simulink library "INT_CnvSet_Trq2Q"  (R2016b)
settings: Solver=VariableStepAuto  StartTime=0.0  StopTime=10.0  RelTol=1e-3
settings Model: Creator=xuxingpei  LastModifiedBy=xuxingpei

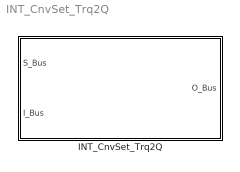
== system INT_CnvSet_Trq2Q ==
  INT_CnvSet_Trq2Q : Subsystem

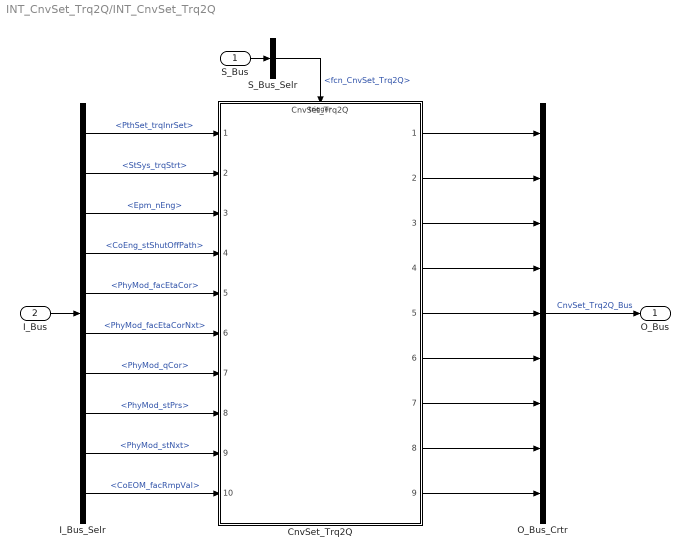
== system INT_CnvSet_Trq2Q/INT_CnvSet_Trq2Q ==
  S_Bus : Inport
  I_Bus : Inport  Port=2
  CnvSet_Trq2Q : ModelReference  ModelNameDialog=CnvSet_Trq2Q  SimulationMode=Normal  ModelReferenceVersion=1.57  TriggerPortName=function  TriggerPortTriggerType=function-call  TriggerPortStatesWhenEnabling=held
  I_Bus_Selr : BusSelector  OutputSignals=PthSet_trqInrSet,StSys_trqStrt,Epm_nEng,CoEng_stShutOffPath,PhyMod_facEtaCor,PhyMod_facEtaCorNxt,PhyMod_qCor,PhyMod_stPrs,PhyMod_stNxt,CoEOM_facRmpVal
  O_Bus_Crtr : BusCreator  Inputs=9
  S_Bus_Selr : BusSelector  OutputSignals=fcn_CnvSet_Trq2Q
  O_Bus : Outport
  wires:
  S_Bus_Selr/1 -> CnvSet_Trq2Q/Trigger  "<fcn_CnvSet_Trq2Q>"
  S_Bus/1 -> S_Bus_Selr/1
  I_Bus/1 -> I_Bus_Selr/1
  I_Bus_Selr/1 -> CnvSet_Trq2Q/1  "<PthSet_trqInrSet>"
  I_Bus_Selr/2 -> CnvSet_Trq2Q/2  "<StSys_trqStrt>"
  I_Bus_Selr/3 -> CnvSet_Trq2Q/3  "<Epm_nEng>"
  I_Bus_Selr/4 -> CnvSet_Trq2Q/4  "<CoEng_stShutOffPath>"
  I_Bus_Selr/5 -> CnvSet_Trq2Q/5  "<PhyMod_facEtaCor>"
  I_Bus_Selr/6 -> CnvSet_Trq2Q/6  "<PhyMod_facEtaCorNxt>"
  I_Bus_Selr/7 -> CnvSet_Trq2Q/7  "<PhyMod_qCor>"
  I_Bus_Selr/8 -> CnvSet_Trq2Q/8  "<PhyMod_stPrs>"
  I_Bus_Selr/9 -> CnvSet_Trq2Q/9  "<PhyMod_stNxt>"
  I_Bus_Selr/10 -> CnvSet_Trq2Q/10  "<CoEOM_facRmpVal>"
  O_Bus_Crtr/1 -> O_Bus/1  "CnvSet_Trq2Q_Bus"
  CnvSet_Trq2Q/1 -> O_Bus_Crtr/1
  CnvSet_Trq2Q/2 -> O_Bus_Crtr/2
  CnvSet_Trq2Q/3 -> O_Bus_Crtr/3
  CnvSet_Trq2Q/4 -> O_Bus_Crtr/4
  CnvSet_Trq2Q/5 -> O_Bus_Crtr/5
  CnvSet_Trq2Q/6 -> O_Bus_Crtr/6
  CnvSet_Trq2Q/7 -> O_Bus_Crtr/7
  CnvSet_Trq2Q/8 -> O_Bus_Crtr/8
  CnvSet_Trq2Q/9 -> O_Bus_Crtr/9
